simulink model "groudstation"  (R2018b)
settings: Solver=VariableStepAuto  StartTime=0.0  StopTime=inf  RelTol=1e-3
undefined symbols (not defined in the file): serial
libraries: instrumentlib x1
settings Model: Creator=E6320  LastModifiedBy=Lakshay Gopalka
settings SFSimCC: SimUseLocalCustomCode=off
settings RTWCC: RTWUseLocalCustomCode=off

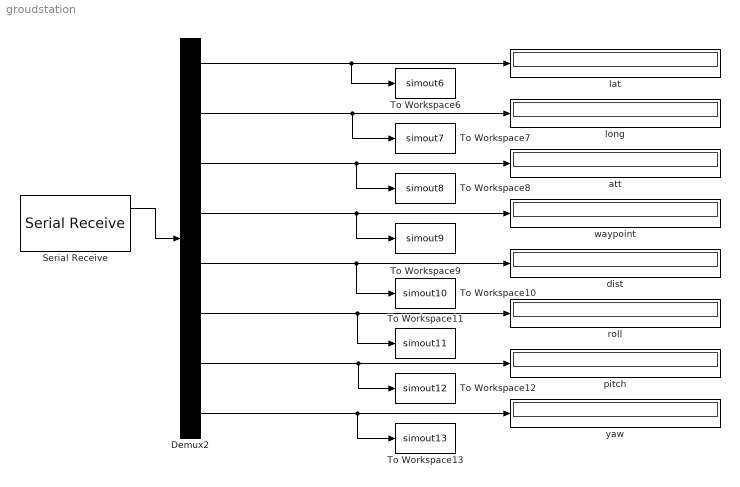
== system groudstation ==
  Demux2 : Demux  Outputs=8
  Serial Receive : instrumentlib/Serial Receive  ComPortMenu=<Please select a port...>  ComPort=COM12  ObjConstructor=serial('COM12');  Terminator=<none>  DataSize="[8  1]"  DataType=single  EnableBlockingMode=off  ActionDataUnavailable=Output last received value  CustomValue=1  SampleTime=0.5
  To Workspace10 : ToWorkspace  VariableName=simout10  SaveFormat=Timeseries  SampleTime=-1
  To Workspace11 : ToWorkspace  VariableName=simout11  SaveFormat=Timeseries  SampleTime=-1
  To Workspace12 : ToWorkspace  VariableName=simout12  SaveFormat=Timeseries  SampleTime=-1
  To Workspace13 : ToWorkspace  VariableName=simout13  SaveFormat=Timeseries  SampleTime=-1
  To Workspace6 : ToWorkspace  VariableName=simout6  SaveFormat=Timeseries  SampleTime=-1
  To Workspace7 : ToWorkspace  VariableName=simout7  SaveFormat=Timeseries  SampleTime=-1
  To Workspace8 : ToWorkspace  VariableName=simout8  SaveFormat=Timeseries  SampleTime=-1
  To Workspace9 : ToWorkspace  VariableName=simout9  SaveFormat=Timeseries  SampleTime=-1
  att : Display
  dist : Display
  lat : Display
  long : Display
  pitch : Display
  roll : Display
  waypoint : Display
  yaw : Display
  wires:
  Serial Receive/1 -> Demux2/1
  Demux2/5 -> To Workspace10/1, dist/1
  Demux2/7 -> To Workspace12/1, pitch/1
  Demux2/1 -> To Workspace6/1, lat/1
  Demux2/2 -> To Workspace7/1, long/1
  Demux2/3 -> To Workspace8/1, att/1
  Demux2/4 -> To Workspace9/1, waypoint/1
  Demux2/6 -> To Workspace11/1, roll/1
  Demux2/8 -> To Workspace13/1, yaw/1
